simulink model "H_inf_implementacion"  (R2023b)
settings: Solver=FixedStepAuto  StartTime=0.0  StopTime=50  RelTol=1e-3  EnableMultiTasking=on
undefined symbols (not defined in the file): h_inf_discreto, T_s
libraries: arduinolib x2
settings Model: ExtModeTrigDuration=2  Creator=Luis Enrique Carmona  LastModifiedBy=chris
settings OptimizationCC: EnhancedBackFolding=on  PassReuseOutputArgsAs=Individual arguments  ZeroExternalMemoryAtStartup=off  ZeroInternalMemoryAtStartup=off  MaxStackSize=64  OptimizeBlockOrder=speed  DifferentSizesBufferReuse=on  OptimizationCustomize=off  EfficientTunableParamExpr=on
settings DebuggingCC: ParameterTunabilityLossMsg=error
settings HardwareCC: ProdBitPerInt=16  ProdBitPerPointer=16  ProdBitPerSizeT=16  ProdBitPerPtrDiffT=16  ProdLargestAtomicFloat=None  ProdWordSize=8  ProdHWDeviceType=Atmel->AVR  UseEmbeddedCoderFeatures=off  UseSimulinkCoderFeatures=off
settings SFSimCC: MATLABDynamicMemAlloc=off
settings RTWCC: Description=Embedded Coder  SystemTargetFile=ert.tlc  HardwareBoard=Arduino Mega 2560  TemplateMakefile=ert_default_tmf  Toolchain=Arduino AVR  BuildConfiguration=Faster Runs  GPUComputeCapability=5.0
settings CodeAppCC: ForceParamTrailComments=on  IgnoreCustomStorageClasses=off  OperatorAnnotations=on  SimulinkDataObjDesc=on  SFDataObjDesc=on  InsertBlockDesc=on
settings ERTTargetCC: SupportContinuousTime=on  SupportNonInlinedSFcns=on  SupportVariableSizeSignals=on  ExtModeTransport=3  ExtModeStaticAlloc=on  ExtModeAutomaticAllocSize=off  ExtModeStaticAllocSize=2048  ExtModeMexFile=ext_xcp  ExtModeIntrfLevel=Level2 - Open

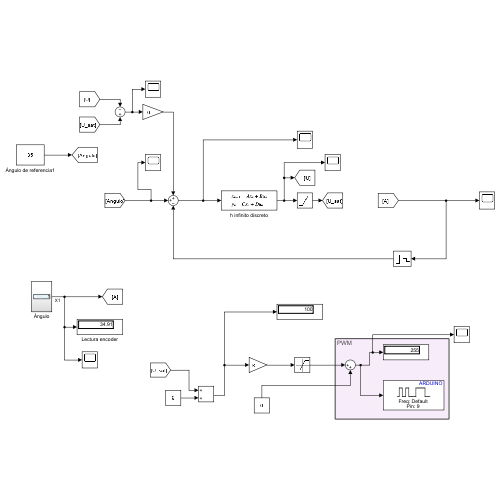
[thumbnail: Simulink's stored preview of the top-level diagram]
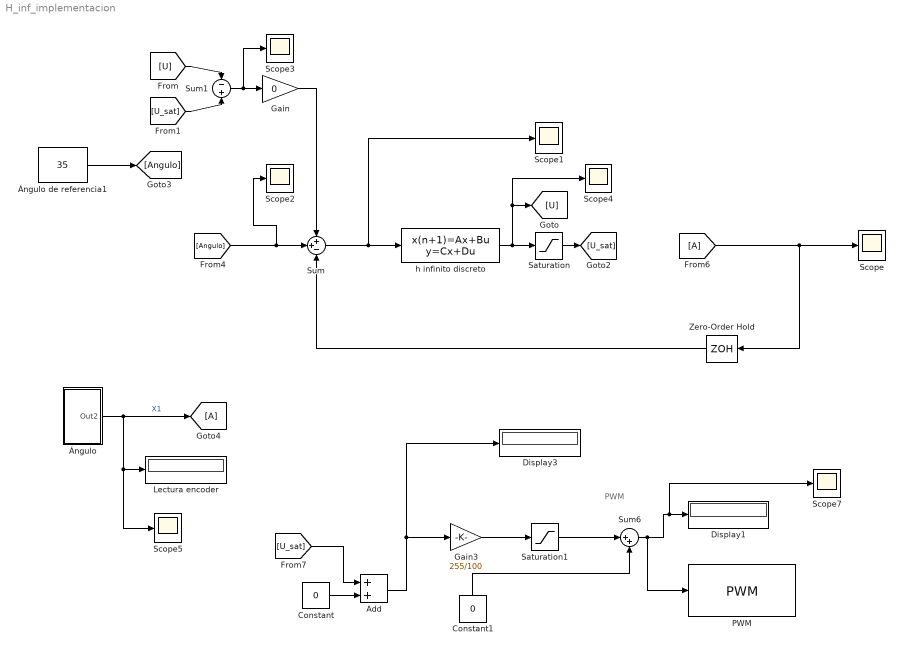
== system H_inf_implementacion ==
  note: PWM
  Add : Sum
  Constant : Constant  Value=0
  Constant1 : Constant  Value=0
  Display1 : Display
  Display3 : Display
  From6 : From
  Gain : Gain  Gain=0
  Gain3 : Gain  Gain=255/100
  Goto4 : Goto
  Lectura encoder : Display
  PWM : arduinolib/PWM  pinNumber=9  frequencyType=Default  desiredFrequency=490.2  achievableFrequency=490.2
  Saturation : Saturate  UpperLimit=100  LowerLimit=0
  Saturation1 : Saturate  UpperLimit=255  LowerLimit=0
  Scope{,1..5,7} (7 alike) : Scope
  Sum : Sum  Inputs=++-
  Sum1 : Sum  Inputs=-|+
  Sum6 : Sum  Inputs=|++
  Zero-Order Hold : ZeroOrderHold  SampleTime=T_s
  h infinito discreto : DiscreteStateSpace  A=h_inf_discreto.A  B=h_inf_discreto.B  C=h_inf_discreto.C  D=0  SampleTime=T_s
  Ángulo : Subsystem
  Ángulo de referencia1 : Constant  Value=35
  wires:
  Zero-Order Hold/1 -> Sum/3
  [Angulo] -> Scope2/1, Sum/2
  From6/1 -> Zero-Order Hold/1, Scope/1
  Sum/1 -> Scope1/1, h infinito discreto/1
  Ángulo de referencia1/1 -> [Angulo]
  [U_sat] -> Add/1
  Sum6/1 -> PWM/1, Scope7/1, Display1/1
  Constant1/1 -> Sum6/2
  Ángulo/1(Out2) -> Goto4/1, Scope5/1, Lectura encoder/1  "X1"
  h infinito discreto/1 -> Saturation/1, [U], Scope4/1
  Add/1 -> Display3/1, Gain3/1
  Constant/1 -> Add/2
  Saturation/1 -> [U_sat]
  [U] -> Sum1/1
  [U_sat] -> Sum1/2
  Sum1/1 -> Scope3/1, Gain/1
  Gain/1 -> Sum/1
  Gain3/1 -> Saturation1/1
  Saturation1/1 -> Sum6/1

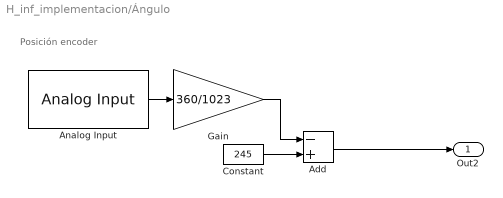
== system H_inf_implementacion/Ángulo ==
  note: Posición encoder
  Add : Sum  Inputs=-+
  Analog Input : arduinolib/Analog Input  pinNumber=0  ReadResultsOnly=off  ConversionTriggerSource=Software  ExternalTriggerType=uint32( 0 )  OutputDataType=uint16  EnableConversionCompleteNotify=off  EnableOuputStatus=off  SampleTime=-1  blockPlatform=arduino
  Constant : Constant  Value=245
  Gain : Gain  Gain=360/1023
  Out2 : Outport
  wires:
  Analog Input/1 -> Gain/1
  Constant/1 -> Add/2
  Gain/1 -> Add/1
  Add/1 -> Out2/1
